simulink subsystem "ideal_alternator"  (R2022b)
settings: Solver=VariableStepAuto  StartTime=0.0  StopTime=10.0  RelTol=1e-3
values from neighbouring files (symbols this model uses):
  alternator = struct()    [Large_engine_params.m]    (also in Small_engine_params.m)
libraries: fl_lib x4, nesl_utility x1, ee_lib x1
settings Model: Creator=wilde  LastModifiedBy=wilde

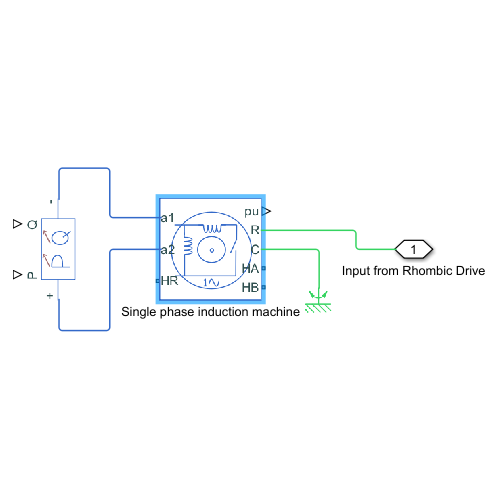
[thumbnail: Simulink's stored preview of the top-level diagram]
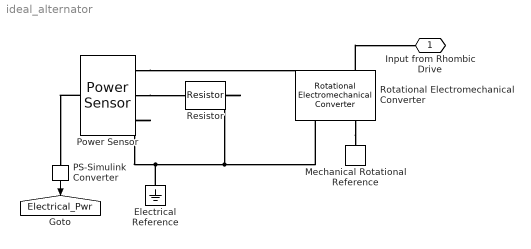
== system ideal_alternator ==
  Electrical Reference : fl_lib/Electrical/Electrical Elements/Electrical Reference
  Mechanical Rotational Reference : fl_lib/Mechanical/Rotational Elements/Mechanical Rotational Reference
  PS-Simulink Converter : nesl_utility/PS-Simulink Converter  PhysicalDomain=network_engine_domain  SubClassName=ps_output  LeftPortType=input  RightPortType=output  PseudoPeriodic=off  Frequencies=[]  VectorFormat=inherit  Unit=inherit  AffineConversion=off
  Power Sensor : ee_lib/Sensors & Transducers/Power Sensor  measurement_type=1  averaging_period=1e-4 s
  Resistor : fl_lib/Electrical/Electrical Elements/Resistor  R=alternator.load.resistance Ohm  i_specify=on  i_priority=High  i=0 A  i_nominal_specify=off  i_nominal_unit=A  i_nominal_value=1  v_specify=on  v_priority=High  v=0 V  v_nominal_specify=off  v_nominal_unit=V  v_nominal_value=1
  Rotational Electromechanical Converter : fl_lib/Electrical/Electrical Elements/Rotational Electromechanical Converter  K=alternator.converter.efficiency V*s/rad  i_specify=off  i_priority=None  i=0 A  i_nominal_specify=off  i_nominal_unit=A  i_nominal_value=1  v_specify=off  v_priority=None  v=0 V  v_nominal_specify=off  v_nominal_unit=V  v_nominal_value=1  t_specify=off  t_priority=None  t=0 N*m  t_nominal_specify=off  t_nominal_unit=N*m  t_nominal_value=1  w_specify=off  w_priority=None  w=0 rad/s  w_nominal_specify=off  w_nominal_unit=rad/s  w_nominal_value=1
  Input from Rhombic Drive : PMIOPort  Side=Left
  tag scope: Electrical_Pwr=global
  wires:
  PS-Simulink Converter/1 -> [Electrical_Pwr]
  connections:
  Electrical Reference/LConn1 -- Power Sensor/LConn3 -- Rotational Electromechanical Converter/RConn1 -- Resistor/RConn1
  Rotational Electromechanical Converter/LConn2 -- Input from Rhombic Drive/RConn1
  Rotational Electromechanical Converter/RConn2 -- Mechanical Rotational Reference/LConn1
  Power Sensor/LConn2 -- Resistor/LConn1
  Power Sensor/RConn1 -- PS-Simulink Converter/LConn1
  Power Sensor/LConn1 -- Rotational Electromechanical Converter/LConn1
